simulink model "performance_specs_block_diagram"  (R2015a)
settings: Solver=ode45  StartTime=0.0  StopTime=10.0  RelTol=1e-3
settings Model: Creator=ayush  LastModifiedBy=ayush

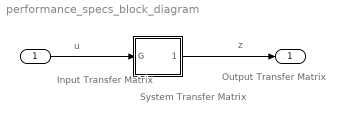
== system performance_specs_block_diagram ==
  note: z
  note: Output
      | Transfer
      | Matrix
  note: u
  note: Input
      | Transfer
      | Matrix
  note: System
      | Transfer
      |  Matrix
  "  " : Inport
  " " : Subsystem
  "     " : Outport
  wires:
  "  "/1 -> " "/1("\t\t\t\t\t\tG")
  " "/1(" ") -> "     "/1

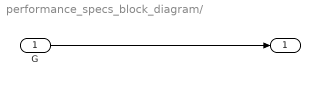
== system performance_specs_block_diagram/  ==
  "\t\t\t\t\t\tG" : Inport
  " " : Outport
  wires:
  "\t\t\t\t\t\tG"/1 -> " "/1
